simulink model "ej2b"  (R2021a)
settings: Solver=VariableStepAuto  StartTime=0.0  StopTime=3000  RelTol=1e-3
libraries: cstblocks x3
settings Model: Creator=franc  LastModifiedBy=franc

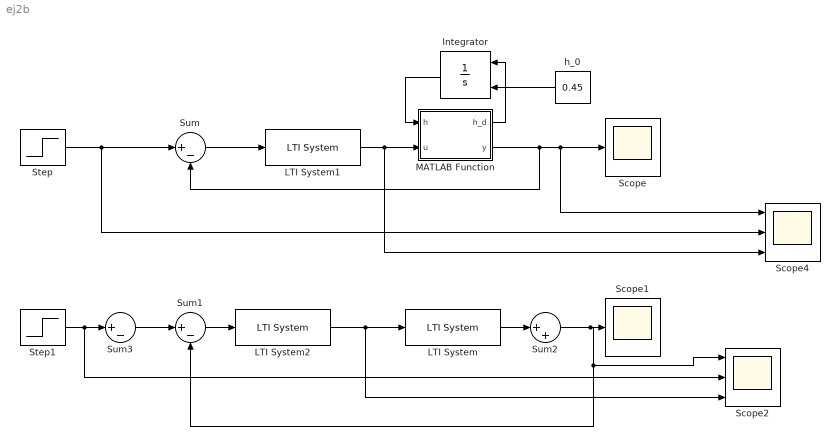
== system ej2b ==
  Integrator : Integrator  InitialConditionSource=external
  LTI System : cstblocks/LTI System  sys=Pmp  IC=[]
  LTI System1 : cstblocks/LTI System  sys=Cs_final  IC=[]
  LTI System2 : cstblocks/LTI System  sys=Cs_final  IC=[]
  MATLAB Function : MATLAB Function  TreatAsAtomicUnit=on
  Scope : Scope
  Scope1 : Scope
  Scope2 : Scope  NumInputPorts=3
  Scope4 : Scope  NumInputPorts=3
  Step : Step  Before=0.45  After=0.4  SampleTime=0
  Step1 : Step  Before=0.45  After=0.4  SampleTime=0
  Sum : Sum  Inputs=|+-
  Sum1 : Sum  Inputs=|+-
  Sum2 : Sum  Inputs=|++
  Sum3 : Sum  Inputs=|+-
  h_0 : Constant  Value=0.45
  wires:
  Step/1 -> Scope4/2, Sum/1
  MATLAB Function/2(y) -> Sum/2, Scope4/1, Scope/1
  MATLAB Function/1(h_d) -> Integrator/1
  Integrator/1 -> MATLAB Function/1(h)
  h_0/1 -> Integrator/2
  LTI System2/1 -> Scope2/3, LTI System/1
  Sum1/1 -> LTI System2/1
  LTI System/1 -> Sum2/1
  Sum2/1 -> Scope2/1, Sum1/2, Scope1/1
  Step1/1 -> Scope2/2, Sum3/1
  Sum3/1 -> Sum1/1
  Sum/1 -> LTI System1/1
  LTI System1/1 -> Scope4/3, MATLAB Function/2(u)

== matlab function ej2b/MATLAB Function ==
  data: h input; h_d output; u input; y output
function [h_d, y] = fcn(h, u)
    g = 9.8;        %En metros sobre segundo cuadrado
    H = 0.9;        %En metros
    L_s = 0.4;      %En metros
    L_i = 0.1;      %En metros
    Q_i = 0.0001333; %Metros cubicos por segundo
    d2 = 10.65e-3;
    A_o = pi * (d2 / 2)^2;

    h_d = (H^2 * (Q_i - A_o * sqrt(2*g*h)*u))/(h^2*(L_s-L_i)^2 + 2*h*L_i*(L_s-L_i)*H+L_i^2*H^2);
    y = h;
end
